simulink model "SimModel"  (R2024b)
settings: Solver=VariableStepAuto  StartTime=0.0  StopTime=10.0  RelTol=1e-3
settings Model: Creator=xinxing  LastModifiedBy=xinxing

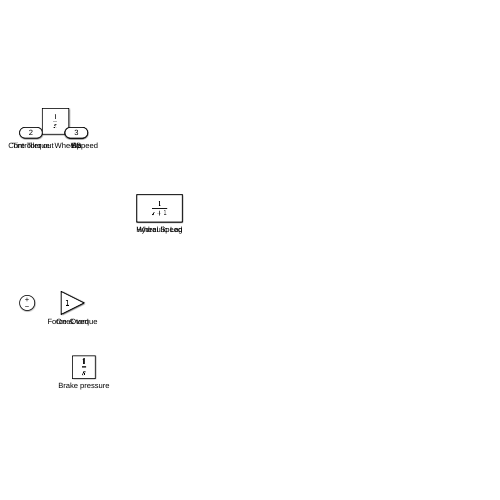
[thumbnail: Simulink's stored preview of the top-level diagram]
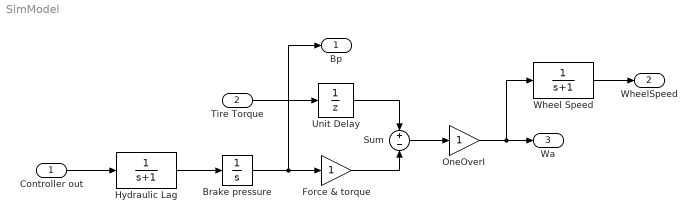
== system SimModel ==
  Controller out : Inport
  Tire Torque : Inport  Port=2
  Brake pressure : Integrator
  Force & torque : Gain
  Hydraulic Lag : TransferFcn  Denominator=[1 1]
  OneOverI : Gain
  Sum : Sum  Inputs=+-
  Unit Delay : UnitDelay  SampleTime=-1  HasFrameUpgradeWarning=on
  Wheel Speed : TransferFcn  Denominator=[1 1]
  Bp : Outport
  WheelSpeed : Outport  Port=2
  Wa : Outport  Port=3
  wires:
  Wheel Speed/1 -> WheelSpeed/1
  Unit Delay/1 -> Sum/1
  Sum/1 -> OneOverI/1
  Brake pressure/1 -> Bp/1, Force & torque/1
  Force & torque/1 -> Sum/2
  Tire Torque/1 -> Unit Delay/1
  Hydraulic Lag/1 -> Brake pressure/1
  OneOverI/1 -> Wheel Speed/1, Wa/1
  Controller out/1 -> Hydraulic Lag/1
